simulink model "hoyas_grandes_i_1_sm_computation"  (R2023b)
settings: Solver=FixedStepDiscrete  StartTime=0.0  StopTime=inf  FixedStep=5e-05  RelTol=1e-3  EnableMultiTasking=on
PostLoadFcn:
  | Ts_Power=50e-6;f=50;R_ac=0.12;L_ac=0.08/(2*pi*50);L1=0.17874;L2=0.07596;L3=0.04321;L4=0.01471;L5=0.04751;L6=0.2054;L7=0.17263;L8=0.14418;L9=0.17697;L10=0.19944;L11=0.18905;L12=0.26987;L13=0.1671;L14=0.16874;L15=0.14664;L16=0.12477;L17=0.14989;L18=0.17217;L19=0.19436; load('PV_prof_norm.mat');
InitFcn:
  | Ts_Power=50e-6;f=50;R_ac=0.12;L_ac=0.08/(2*pi*50);L1=0.17874;L2=0.07596;L3=0.04321;L4=0.01471;L5=0.04751;L6=0.2054;L7=0.17263;L8=0.14418;L9=0.17697;L10=0.19944;L11=0.18905;L12=0.26987;L13=0.1671;L14=0.16874;L15=0.14664;L16=0.12477;L17=0.14989;L18=0.17217;L19=0.19436; load('PV_prof_norm.mat');
undefined symbols (not defined in the file or in its folder): D11, Delta, L, X_ac
libraries: spsVoltageMeasurementLib x84, spsCurrentMeasurementLib x75, rtlab x39, spsThreePhaseSeriesRLCBranchLib x38, spsGroundLib x28, powerlib_extras x25, spsThreePhaseDynamicLoadLib x19, eeGeneralControl x4, rteventslib x4, opal_lib x3, spsThreePhasePISectionLineLib x2, spsThreePhaseTransformerTwoWindingsLib x2
(part 1 of 4)
Description:
  | Model of a simple control system for use iin training.
settings Model: Creator=Paul Baracos  LastModifiedBy=depto
settings SolverCC: AlgebraicLoopSolver=TrustRegion
settings DataIOCC: LimitDataPoints=on  SaveFormat=Array  SignalLoggingSaveFormat=ModelDataLogs  SaveOutput=off  SaveTime=off  ReturnWorkspaceOutputs=off  SignalLoggingName=sigsOut
settings OptimizationCC: BlockReduction=off  BooleanDataType=off  OptimizeBlockIOStorage=off  BufferReuse=off  ExpressionFolding=off  LocalBlockOutputs=off  InitFltsAndDblsToZero=on  LifeSpan=inf
settings DebuggingCC: SaveWithParameterizedLinksMsg=none  UnderspecifiedInitializationDetection=Classic  MergeDetectMultiDrivingBlocksExec=none  SignalResolutionControl=TryResolveAllWithWarning  MultiTaskDSMMsg=warning  MultiTaskCondExecSysMsg=none  FcnCallInpInsideContextMsg=warning  UnconnectedInputMsg=warning  UnconnectedOutputMsg=warning  UnconnectedLineMsg=warning  SFUnexpectedBacktrackingDiag=warning  SFNoUnconditionalDefaultTransitionDiag=warning  SFExecutionAtInitializationDiag=none  ArithmeticOperatorsInVariantConditions=warning
settings HardwareCC: ProdBitPerPointer=32  ProdBitPerSizeT=32  ProdBitPerPtrDiffT=32  ProdLargestAtomicFloat=None  ProdIntDivRoundTo=Undefined  ProdEndianess=Unspecified  ProdWordSize=32  ProdHWDeviceType=32-bit Generic  TargetUnknown=on
settings ModelReferenceCC: EnableRefExpFcnMdlSchedulingChecks=on  PropagateSignalLabelsOutOfModel=off
settings SFSimCC: SimUseLocalCustomCode=off  CustomCodeUndefinedFunction=UseInterfaceOnly
settings RTWCC: GenCodeOnly=on  RTWUseLocalCustomCode=off
settings CodeAppCC: StateflowObjectComments=on
settings GRTTargetCC: TargetFcnLib=ansi_tfl_tmw.mat  TargetLangStandard=C89/C90 (ANSI)  CombineOutputUpdateFcns=off  GRTInterface=on
settings ConfigComp: CovMetricSettings=dw  CovSaveCumulativeToWorkspaceVar=on  CovSaveSingleToWorkspaceVar=on  CovExternalEMLEnable=off

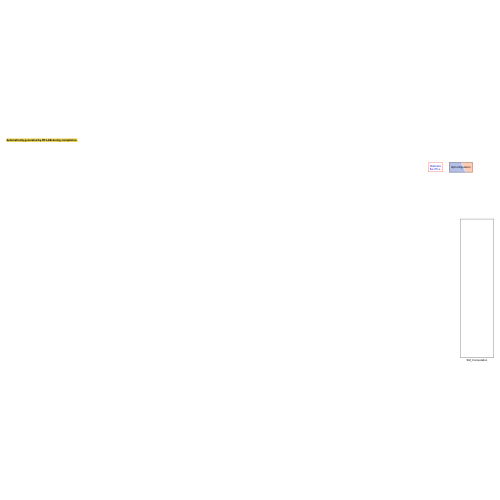
[thumbnail: Simulink's stored preview of the top-level diagram]
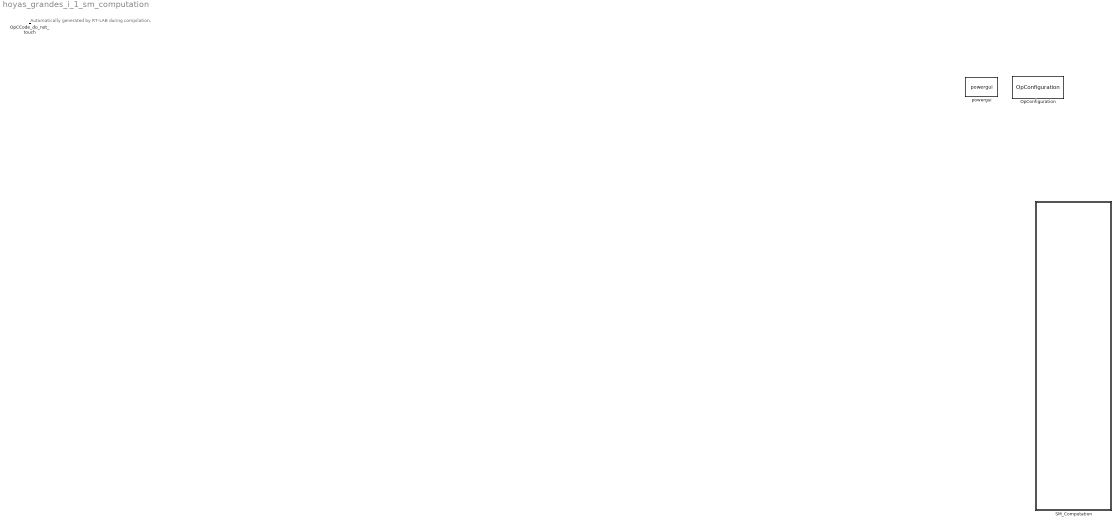
== system hoyas_grandes_i_1_sm_computation ==
  note: Automatically generated by RT-LAB during compilation.
  OpCCode_do_not_touch : opal_lib/Communication/OpCCode  SystemSampleTime=-1  VariantActivationTime=update diagram  AllowFlexibleInterface=on  Latency=0  AutoFrameSizeCalculation=off
  OpConfiguration : rtlab/Miscellaneous/OpConfiguration  Page=Target platform  AddFileBeforeLoad=DatosConstant.mat=binary  AddTargetQnx=off  AddTargetRH=on  AddTargetWin=off  AddTargetPetalinux=on  AddTargetOpalRT=on
      settings: SourceProductName=RT-LAB
  SM_Computation : Subsystem
  powergui : spspowerguiLib/powergui  SimulationMode=Discrete  SampleTime=5e-05  frequency=60  Iterations=50  frequencyindice=50  Pbase=100e6  ErrMax=1e-4  UnitsV=kV  UnitsW=MW  buscounter=0  FunctionMessages=off  echomessages=off  EnableUseOfTLC=off  CurrentSourceSwitches=off  DisableSnubberDevices=off  DisableRonSwitches=off  DisableVfSwitches=off  DisplayEquations=off  AutomaticDiscreteSolvers=off  SolverType=Tustin  Interpol=off  ExternalGateDelay=off  methode=off  Ts=100  x0status=blocks  SPID=off  SwTol=0  HookPort=off  NonlinearTolerance=1e-4  nMaxIteration=100  ContinueOnMaxIteration=off  RestoreLinks=warning  ResistiveCurrentMeasurement=off  Frange=[0:2:500]  Ylog=off  Xlog=on  ShowGrid=off  save=off  variable=ZData  structure=0  ZoomFFT=off  StartTime=0.0  cycles=1  DisplayStyle=1  fundamental=60  FreqAxis=off  MaxFrequency=1000  frequencyindicesteady=1  RmsSteady=1  display=off

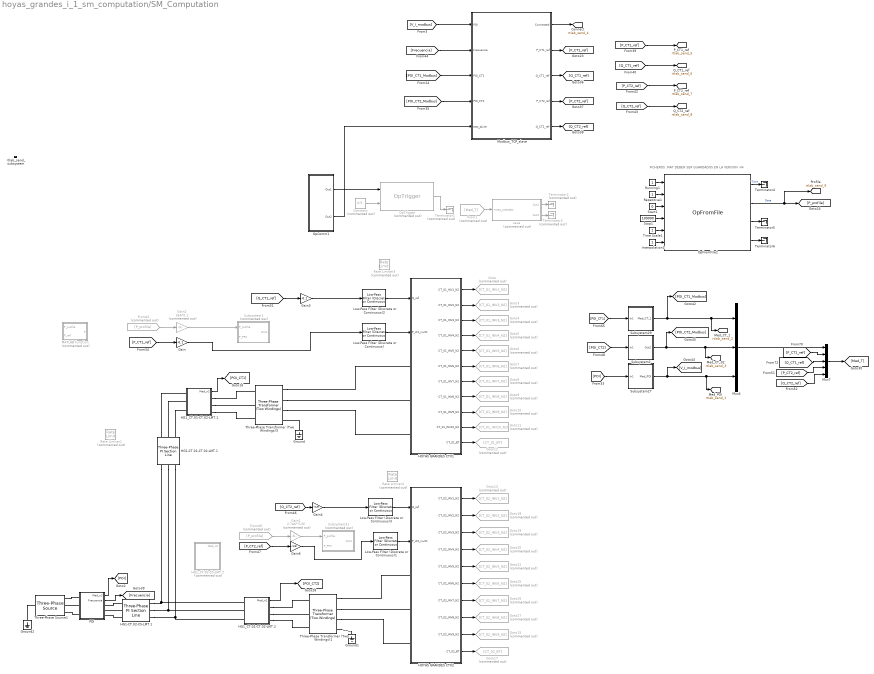
== system hoyas_grandes_i_1_sm_computation/SM_Computation ==
  note: FICHEROS .MAT DEBEN SER GUARDADOS EN LA VERSION -V4
  Constant : Constant  Commented=on  Value=0.5
  From1 : From  Commented=on  GotoTag=Med_T
  From41 : From  Commented=on  GotoTag=P_profile
  From49 : From  Commented=on  GotoTag=P_profile
  Gain : Gain  Gain=-0.1
  Gain1 : Gain  Commented=on  Gain=2.7e6*(1/9)
  Gain2 : Gain  Commented=on  Gain=3e6*0.1
  Gain3 : Gain  Gain=-0.1
  Gain4 : Gain  Gain=-(1/9)
  Gain6 : Gain  Gain=-(1/9)
  Goto : Goto  Commented=on  GotoTag=CT_01_INV1_N2
  Goto10 : Goto  Commented=on  GotoTag=CT_01_INV9_N2
  Goto11 : Goto  Commented=on  GotoTag=CT_01_INV10_N2
  Goto12 : Goto  Commented=on  GotoTag=CT_01_BT
  Goto13 : Goto  Commented=on  GotoTag=CT_02_INV1_N2
  Goto15 : Goto  Commented=on  GotoTag=CT_02_INV9_N2
  Goto17 : Goto  Commented=on  GotoTag=CT_02_BT
  Goto18 : Goto  Commented=on  GotoTag=CT_02_INV2_N2
  Goto19 : Goto  Commented=on  GotoTag=CT_02_INV3_N2
  Goto20 : Goto  Commented=on  GotoTag=CT_02_INV4_N2
  Goto22 : Goto  Commented=on  GotoTag=CT_02_INV5_N2
  Goto25 : Goto  Commented=on  GotoTag=CT_02_INV6_N2
  Goto26 : Goto  Commented=on  GotoTag=CT_02_INV7_N2
  Goto27 : Goto  Commented=on  GotoTag=CT_02_INV8_N2
  Goto3 : Goto  Commented=on  GotoTag=CT_01_INV2_N2
  Goto4 : Goto  Commented=on  GotoTag=CT_01_INV3_N2
  Goto5 : Goto  Commented=on  GotoTag=CT_01_INV4_N2
  Goto6 : Goto  Commented=on  GotoTag=CT_01_INV5_N2
  Goto7 : Goto  Commented=on  GotoTag=CT_01_INV6_N2
  Goto8 : Goto  Commented=on  GotoTag=CT_01_INV7_N2
  Goto9 : Goto  Commented=on  GotoTag=CT_01_INV8_N2
  Ground : spsGroundLib/Ground  LConnTagsString=a
  Ground1 : spsGroundLib/Ground  LConnTagsString=a
  Ground2 : spsGroundLib/Ground  LConnTagsString=a
  HG1-CT.01-CT.02-LMT.1 : spsThreePhasePISectionLineLib/Three-Phase PI Section Line  LConnTagsString=a|b|c  RConnTagsString=A|B|C  Length=0.613  Frequency=50  Resistances=[ 0.206 0.206]  Inductances="[ 0.115/(2*pi*f)  0.115/(2*pi*f)]"  Capacitances=[0.235e-6 0.235e-6]
  HG1-CT.02-CS-LMT.1 : spsThreePhasePISectionLineLib/Three-Phase PI Section Line  LConnTagsString=a|b|c  RConnTagsString=A|B|C  Length=0.153  Frequency=50  Resistances=[ 0.206 0.206]  Inductances="[ 0.115/(2*pi*f)  0.115/(2*pi*f)]"  Capacitances=[0.235e-6 0.235e-6]
  HG1_CT.01-CT.02-LMT.1 : Subsystem
  HG1_CT.01-CT.02-LMT.2 : Subsystem
  HG1_CT.02-CS-LMT.2 : Subsystem  Commented=on
  HOYAS GRANDES CT01 : Subsystem
  HOYAS GRANDES CT02 : Subsystem
  Interpolation1 : Constant
  Low-Pass Filter (Discrete or Continuous){,1..3} (4 alike) : eeGeneralControl/Low-Pass Filter (Discrete or Continuous)  K=1  T=0.03575  B=inf  A=-inf  init_option=Inherited from block input  x0=0  Ts=-1
  MATLAB Function : MATLAB Function  Commented=on  TreatAsAtomicUnit=on
  Modbus_TCP_slave : Subsystem
  Mux4 : Mux  Inputs=3
  Mux7 : Mux  Inputs=5
  OpComm1 : Subsystem
      mask init:
      | opmaskdisplay('maskdisplay_block',gcb,'disp(''OpComm'')');
      mask Display:
      | patch([0 0.5 0.7 0],[1 1 0 0],[0.7 0.75 0.9]);
      | patch([1 0.53 0.73 1],[1 1 0 0],[1 0.8 0.7]);
      | plot([0 0 1 1 0],[0 1 1 0 0]);
      | disp('OpComm')
  OpFromFile2 : rtlab/DataLogging/OpFromFile  filename_mode=Static (same filename all the time)  reload_mode=Next time model is paused (Real-Time)  init_file_id=0  filename=PV_prof_norm.mat  rtpath='./'  nrtpath='.\'  sample_time=0
      settings: SourceProductName=RT-LAB
  OpTrigger : rtlab/DataLogging/OpTrigger  Commented=on  Trig_Type=RISING EDGE  Trig_Offset=0  Acq_Group=28
      settings: SourceProductName=RT-LAB
  POI : Subsystem
  Rate Limiter1 : RateLimiter  Commented=on  RisingSlewLimit=250000*3.5  FallingSlewLimit=-250000*3.5  SampleTimeMode=inherited
  Rate Limiter3 : RateLimiter  Commented=on  RisingSlewLimit=250000*2  FallingSlewLimit=-250000*2  SampleTimeMode=inherited
  Rate Limiter4 : RateLimiter  Commented=on  RisingSlewLimit=250000*2  FallingSlewLimit=-250000*2  SampleTimeMode=inherited
  Repetitive1 : Constant
  Running1 : Constant
  Start1 : Constant  Value=0
  Stop1 : Constant  Value=100000
  Subsystem1 : Subsystem  Commented=on
  Subsystem2 : Subsystem
  Subsystem27 : Subsystem
  Subsystem29 : Subsystem
  Subsystem31 : Subsystem  Commented=on
  Terminator1 : Terminator  Commented=on
  Terminator2 : Terminator  Commented=on
  Terminator3 : Terminator  Commented=on
  Terminator4 : Terminator
  Terminator5 : Terminator
  Terminator6 : Terminator
  Three-Phase Transformer (Two Windings)1 : spsThreePhaseTransformerTwoWindingsLib/Three-Phase Transformer (Two Windings)  Winding1Connection=Delta (D11)  Winding2Connection=Yn  CoreType=Three single-phase transformers  SetSaturation=off  Hysteresis=off  DataFile='hysteresis'  SetInitialFlux=off  Measurements=None  UNITS=pu  NominalPower=[ 3e6 , 50 ]  Winding1=[ 20e3 , 0.0073/2 , 0.0596/2 ]  Winding2=[ 800 , 0.0073/2, 0.0596/2]  Rm=4.7695e3  Lm=4.7695e3  L0=0.5  Saturation=[ 0,0 ; 0.0024,1.2 ; 1.0,1.52 ]  InitialFluxes=[ 0.8 , -0.8 , 0.7 ]  BreakLoop=off  DiscreteSolver=Trapezoidal iterative  DataType=off  TransfoNumber=1
  Three-Phase Transformer (Two Windings)3 : spsThreePhaseTransformerTwoWindingsLib/Three-Phase Transformer (Two Windings)  Winding1Connection=Delta (D11)  Winding2Connection=Yn  CoreType=Three single-phase transformers  SetSaturation=off  Hysteresis=off  DataFile='hysteresis'  SetInitialFlux=off  Measurements=None  UNITS=pu  NominalPower=[ 3e6 , 50 ]  Winding1=[ 20e3 , 0.0073/2 , 0.0596/2 ]  Winding2=[ 800 , 0.0073/2, 0.0596/2]  Rm=4.7695e3  Lm=4.7695e3  L0=0.5  Saturation=[ 0,0 ; 0.0024,1.2 ; 1.0,1.52 ]  InitialFluxes=[ 0.8 , -0.8 , 0.7 ]  BreakLoop=off  DiscreteSolver=Trapezoidal iterative  DataType=off  TransfoNumber=1
  Three-Phase Source1 : spsThreePhaseSourceLib/Three-Phase Source  InternalConnection=Yn  VoltagePhases=off  Voltage=20e3  PhaseAngle=0  Voltage_phases=[25e3 25e3 25e3]/sqrt(3)  PhaseAngles_phases=[0 -120 +120]  Frequency=50  NonIdealSource=on  SpecifyImpedance=on  Resistance=0.8929  Inductance=16.58e-3  ShortCircuitLevel=150.486e6  BaseVoltage=20000  XRratio=3.37  BusType=swing  Pref=10e3  Qref=0  Prefabc=[10e3, 10e3, 10e3]  Qrefabc=[0, 0, 0]  Qmin=-inf  Qmax=inf
  Time Scale1 : Constant
  rtlab_send_subsystem : Subsystem  Priority=-100
      mask Display: text(0,0,'');
  save : Subsystem  Commented=on
  tag scope: rtlab_send_1=global, rtlab_send_2=global, rtlab_send_3=global, rtlab_send_4=global, rtlab_send_5=global, rtlab_send_6=global, rtlab_send_7=global, rtlab_send_8=global, rtlab_send_9=global
  wires:
  [P_CT1_ref] -> Gain/1
  Interpolation1/1 -> OpFromFile2/6
  Repetitive1/1 -> OpFromFile2/2
  HOYAS GRANDES CT02/9(CT_02_INV9_N2) -> Goto15/1
  Gain3/1 -> Low-Pass Filter (Discrete or Continuous)2/1
  OpFromFile2/3 -> Terminator5/1
  Low-Pass Filter (Discrete or Continuous)/1 -> HOYAS GRANDES CT01/2(P_ct1_inv01)
  OpFromFile2/1 -> Terminator4/1  "Time"
  Stop1/1 -> OpFromFile2/4
  HOYAS GRANDES CT01/7(CT_01_INV7_N2) -> Goto8/1
  POI/2(Frecuencia) -> [Frecuencia]
  Running1/1 -> OpFromFile2/1
  [P_CT2_ref] -> Mux7/4
  HOYAS GRANDES CT01/10(CT_01_INV10_N2) -> Goto11/1
  HOYAS GRANDES CT02/8(CT_02_INV8_N2) -> Goto27/1
  OpFromFile2/2 -> [rtlab_send_9], [P_profile]  "Data"
  HG1_CT.01-CT.02-LMT.2/1(Med_n2) -> [POI_CT2]
  OpFromFile2/4 -> Terminator6/1
  HOYAS GRANDES CT01/2(CT_01_INV2_N2) -> Goto3/1
  Start1/1 -> OpFromFile2/3
  [P_CT1_ref] -> Mux7/2
  HOYAS GRANDES CT01/11(CT_01_BT) -> Goto12/1
  HOYAS GRANDES CT02/7(CT_02_INV7_N2) -> Goto26/1
  Time Scale1/1 -> OpFromFile2/5
  Mux7/1 -> [Med_T]
  Subsystem27/1(Med_POI) -> [rtlab_send_1], Mux4/3, [V_I_modbus]
  HOYAS GRANDES CT01/9(CT_01_INV9_N2) -> Goto10/1
  Low-Pass Filter (Discrete or Continuous)1/1 -> HOYAS GRANDES CT02/2(P_ct2_inv01)
  HOYAS GRANDES CT02/2(CT_02_INV2_N2) -> Goto18/1
  HOYAS GRANDES CT01/1(CT_01_INV1_N2) -> Goto/1
  HG1_CT.01-CT.02-LMT.1/1(Med_n2) -> [POI_CT1]
  HOYAS GRANDES CT01/8(CT_01_INV8_N2) -> Goto9/1
  [P_CT2_ref] -> Gain6/1
  From49/1 -> Gain1/1
  HOYAS GRANDES CT01/4(CT_01_INV4_N2) -> Goto5/1
  HOYAS GRANDES CT02/6(CT_02_INV6_N2) -> Goto25/1
  HOYAS GRANDES CT01/5(CT_01_INV5_N2) -> Goto6/1
  HOYAS GRANDES CT02/10(CT_02_BT) -> Goto17/1
  HOYAS GRANDES CT02/5(CT_02_INV5_N2) -> Goto22/1
  HOYAS GRANDES CT02/4(CT_02_INV4_N2) -> Goto20/1
  HOYAS GRANDES CT02/1(CT_02_INV1_N2) -> Goto13/1
  [Q_CT1_ref] -> Mux7/3
  [POI_CT2] -> Subsystem2/1(In1)
  From41/1 -> Gain2/1
  Subsystem2/1(Out2) -> [rtlab_send_3], Mux4/2, [POI_CT2_Modbus]
  Gain4/1 -> Low-Pass Filter (Discrete or Continuous)3/1
  Mux4/1 -> Mux7/1
  HOYAS GRANDES CT01/6(CT_01_INV6_N2) -> Goto7/1
  Subsystem29/1(Med_CT_1) -> [POI_CT1_Modbus], [rtlab_send_2], Mux4/1
  [Q_CT1_ref] -> Gain3/1
  Low-Pass Filter (Discrete or Continuous)2/1 -> HOYAS GRANDES CT01/1(Q_ref)
  [Q_CT2_ref] -> Mux7/5
  [POI_CT1] -> Subsystem29/1(In1)
  POI/1(Med_n2) -> [POI]
  [Q_CT2_ref] -> Gain4/1
  HOYAS GRANDES CT01/3(CT_01_INV3_N2) -> Goto4/1
  OpTrigger/1 -> Terminator1/1
  HOYAS GRANDES CT02/3(CT_02_INV3_N2) -> Goto19/1
  [POI] -> Subsystem27/1(In1)
  Low-Pass Filter (Discrete or Continuous)3/1 -> HOYAS GRANDES CT02/1(Q_ref)
  OpComm1/1(Out1) -> OpTrigger/1
  From1/1 -> save/1(meas_tratadas)
  save/1(Out1) -> Terminator2/1
  Constant/1 -> OpTrigger/2
  save/2(Out2) -> Terminator3/1
  Modbus_TCP_slave/5(Q_CT2_ref) -> [Q_CT2_ref]
  [POI_CT2_Modbus] -> Modbus_TCP_slave/4(POI_CT2)
  Modbus_TCP_slave/3(Q_CT1_ref) -> [Q_CT1_ref]
  [POI_CT1_Modbus] -> Modbus_TCP_slave/3(POI_CT1)
  Modbus_TCP_slave/4(P_CT2_ref) -> [P_CT2_ref]
  Modbus_TCP_slave/1(Connected) -> [rtlab_send_4]
  [V_I_modbus] -> Modbus_TCP_slave/1(POI)
  [Frecuencia] -> Modbus_TCP_slave/2(Frecuencia)
  Modbus_TCP_slave/2(P_CT1_ref) -> [P_CT1_ref]
  [Q_CT2_ref] -> [rtlab_send_8]
  [P_CT2_ref] -> [rtlab_send_7]
  [Q_CT1_ref] -> [rtlab_send_6]
  [P_CT1_ref] -> [rtlab_send_5]
  Gain1/1 -> Subsystem31/1(P_profile)
  Gain6/1 -> Low-Pass Filter (Discrete or Continuous)1/1
  Gain2/1 -> Subsystem1/1(P_profile)
  Gain/1 -> Low-Pass Filter (Discrete or Continuous)/1
  OpComm1/2(Out2) -> Modbus_TCP_slave/5(test_JAvier)
  connections:
  Three-Phase Transformer (Two Windings)1/RConn4 -- Ground1/LConn1
  HG1-CT.01-CT.02-LMT.1/RConn3 -- HG1_CT.01-CT.02-LMT.1/LConn3
  Ground/LConn1 -- Three-Phase Transformer (Two Windings)3/RConn4
  Three-Phase Transformer (Two Windings)3/RConn3 -- HOYAS GRANDES CT01/LConn3
  Three-Phase Transformer (Two Windings)1/RConn3 -- HOYAS GRANDES CT02/LConn3
  HG1-CT.01-CT.02-LMT.1/RConn2 -- HG1_CT.01-CT.02-LMT.1/LConn2
  HG1-CT.02-CS-LMT.1/LConn1 -- POI/RConn1
  HG1_CT.01-CT.02-LMT.1/RConn3 -- Three-Phase Transformer (Two Windings)3/LConn3
  POI/LConn1 -- Three-Phase Source1/RConn1
  Three-Phase Transformer (Two Windings)3/RConn2 -- HOYAS GRANDES CT01/LConn2
  Three-Phase Transformer (Two Windings)1/RConn1 -- HOYAS GRANDES CT02/LConn1
  HG1_CT.01-CT.02-LMT.2/RConn2 -- Three-Phase Transformer (Two Windings)1/LConn2
  HG1_CT.01-CT.02-LMT.1/RConn2 -- Three-Phase Transformer (Two Windings)3/LConn2
  HG1-CT.02-CS-LMT.1/RConn3 -- HG1_CT.01-CT.02-LMT.2/LConn3 -- HG1-CT.01-CT.02-LMT.1/LConn3
  HG1_CT.01-CT.02-LMT.2/RConn1 -- Three-Phase Transformer (Two Windings)1/LConn1
  HG1-CT.02-CS-LMT.1/RConn1 -- HG1_CT.01-CT.02-LMT.2/LConn1 -- HG1-CT.01-CT.02-LMT.1/LConn1
  HG1-CT.02-CS-LMT.1/RConn2 -- HG1_CT.01-CT.02-LMT.2/LConn2 -- HG1-CT.01-CT.02-LMT.1/LConn2
  Three-Phase Transformer (Two Windings)3/RConn1 -- HOYAS GRANDES CT01/LConn1
  Ground2/LConn1 -- Three-Phase Source1/LConn1
  HG1-CT.02-CS-LMT.1/LConn3 -- POI/RConn3
  HG1_CT.01-CT.02-LMT.2/RConn3 -- Three-Phase Transformer (Two Windings)1/LConn3
  POI/LConn2 -- Three-Phase Source1/RConn2
  POI/LConn3 -- Three-Phase Source1/RConn3
  HG1_CT.01-CT.02-LMT.1/RConn1 -- Three-Phase Transformer (Two Windings)3/LConn1
  HG1-CT.02-CS-LMT.1/LConn2 -- POI/RConn2
  HG1-CT.01-CT.02-LMT.1/RConn1 -- HG1_CT.01-CT.02-LMT.1/LConn1
  Three-Phase Transformer (Two Windings)1/RConn2 -- HOYAS GRANDES CT02/LConn2

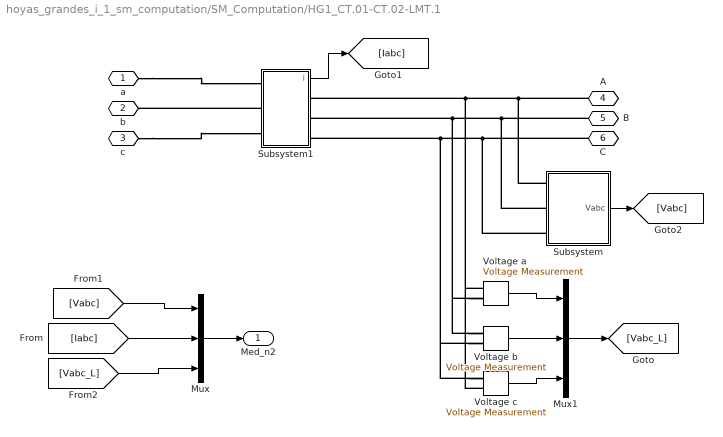
== system hoyas_grandes_i_1_sm_computation/SM_Computation/HG1_CT.01-CT.02-LMT.1 ==
  Mux : Mux  Inputs=3
  Mux1 : Mux  Inputs=3
  Subsystem : Subsystem
  Subsystem1 : Subsystem
  Voltage a : spsVoltageMeasurementLib/Voltage Measurement  PhasorSimulation=off  OutputType=Complex  PSBequivalent=0
  Voltage b : spsVoltageMeasurementLib/Voltage Measurement  PhasorSimulation=off  OutputType=Complex  PSBequivalent=0
  Voltage c : spsVoltageMeasurementLib/Voltage Measurement  PhasorSimulation=off  OutputType=Complex  PSBequivalent=0
  a : PMIOPort  Side=Right
  b : PMIOPort  Port=2  Side=Right
  c : PMIOPort  Port=3  Side=Right
  A : PMIOPort  Port=4  Side=Left
  B : PMIOPort  Port=5  Side=Left
  C : PMIOPort  Port=6  Side=Left
  Med_n2 : Outport
  wires:
  Subsystem1/1(i) -> [Iabc]
  [Vabc] -> Mux/1
  [Iabc] -> Mux/2
  Mux/1 -> Med_n2/1
  Voltage a/1 -> Mux1/1
  Voltage b/1 -> Mux1/2
  Voltage c/1 -> Mux1/3
  Mux1/1 -> [Vabc_L]
  Subsystem/1(Vabc) -> [Vabc]
  [Vabc_L] -> Mux/3
  connections:
  B/RConn1 -- Subsystem/LConn2 -- Voltage b/LConn1 -- Voltage a/LConn2 -- Subsystem1/RConn2
  A/RConn1 -- Subsystem/LConn1 -- Voltage a/LConn1 -- Voltage c/LConn2 -- Subsystem1/RConn1
  C/RConn1 -- Subsystem/LConn3 -- Voltage c/LConn1 -- Voltage b/LConn2 -- Subsystem1/RConn3
  c/RConn1 -- Subsystem1/LConn3
  Subsystem1/LConn2 -- b/RConn1
  a/RConn1 -- Subsystem1/LConn1

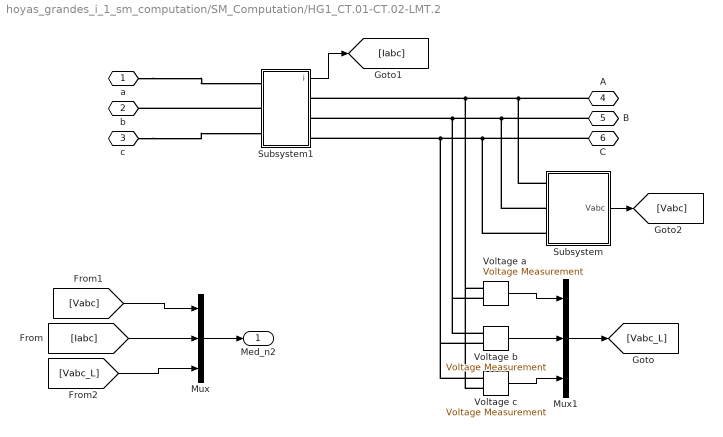
== system hoyas_grandes_i_1_sm_computation/SM_Computation/HG1_CT.01-CT.02-LMT.2 ==
  Mux : Mux  Inputs=3
  Mux1 : Mux  Inputs=3
  Subsystem : Subsystem
  Subsystem1 : Subsystem
  Voltage a : spsVoltageMeasurementLib/Voltage Measurement  PhasorSimulation=off  OutputType=Complex  PSBequivalent=0
  Voltage b : spsVoltageMeasurementLib/Voltage Measurement  PhasorSimulation=off  OutputType=Complex  PSBequivalent=0
  Voltage c : spsVoltageMeasurementLib/Voltage Measurement  PhasorSimulation=off  OutputType=Complex  PSBequivalent=0
  a : PMIOPort  Side=Right
  b : PMIOPort  Port=2  Side=Right
  c : PMIOPort  Port=3  Side=Right
  A : PMIOPort  Port=4  Side=Left
  B : PMIOPort  Port=5  Side=Left
  C : PMIOPort  Port=6  Side=Left
  Med_n2 : Outport
  wires:
  [Vabc_L] -> Mux/3
  Subsystem/1(Vabc) -> [Vabc]
  Mux1/1 -> [Vabc_L]
  Voltage c/1 -> Mux1/3
  Voltage b/1 -> Mux1/2
  Voltage a/1 -> Mux1/1
  Mux/1 -> Med_n2/1
  [Iabc] -> Mux/2
  [Vabc] -> Mux/1
  Subsystem1/1(i) -> [Iabc]
  connections:
  a/RConn1 -- Subsystem1/LConn1
  Subsystem1/LConn2 -- b/RConn1
  c/RConn1 -- Subsystem1/LConn3
  Subsystem/LConn3 -- C/RConn1 -- Subsystem1/RConn3 -- Voltage b/LConn2 -- Voltage c/LConn1
  Subsystem/LConn1 -- A/RConn1 -- Subsystem1/RConn1 -- Voltage c/LConn2 -- Voltage a/LConn1
  Subsystem/LConn2 -- B/RConn1 -- Subsystem1/RConn2 -- Voltage a/LConn2 -- Voltage b/LConn1

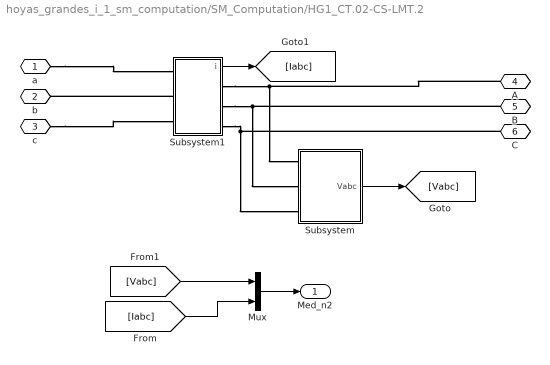
== system hoyas_grandes_i_1_sm_computation/SM_Computation/HG1_CT.02-CS-LMT.2 ==
  Mux : Mux  Inputs=2
  Subsystem : Subsystem
  Subsystem1 : Subsystem
  a : PMIOPort  Side=Right
  b : PMIOPort  Port=2  Side=Right
  c : PMIOPort  Port=3  Side=Right
  A : PMIOPort  Port=4  Side=Left
  B : PMIOPort  Port=5  Side=Left
  C : PMIOPort  Port=6  Side=Left
  Med_n2 : Outport
  wires:
  Subsystem/1(Vabc) -> [Vabc]
  Subsystem1/1(i) -> [Iabc]
  [Vabc] -> Mux/1
  [Iabc] -> Mux/2
  Mux/1 -> Med_n2/1
  connections:
  Subsystem1/RConn2 -- B/RConn1 -- Subsystem/LConn2
  Subsystem1/RConn1 -- A/RConn1 -- Subsystem/LConn1
  Subsystem1/RConn3 -- C/RConn1 -- Subsystem/LConn3
  c/RConn1 -- Subsystem1/LConn3
  Subsystem1/LConn2 -- b/RConn1
  a/RConn1 -- Subsystem1/LConn1

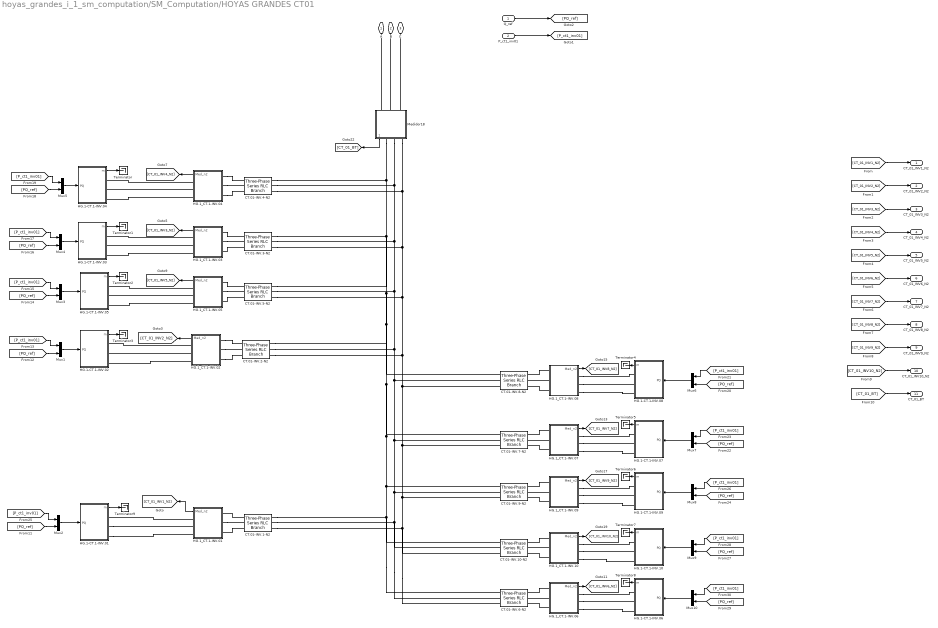
== system hoyas_grandes_i_1_sm_computation/SM_Computation/HOYAS GRANDES CT01 ==
  Q_ref : Inport
  P_ct1_inv01 : Inport  Port=2
  CT.01-INV.1-N2 : spsThreePhaseSeriesRLCBranchLib/Three-Phase Series RLC Branch  LConnTagsString=A|B|C  RConnTagsString=A|B|C  BranchType=RL  Resistance=R_ac*L1  Inductance=L_ac*L1  Capacitance=1e-6  Measurements=None
  CT.01-INV.10-N2 : spsThreePhaseSeriesRLCBranchLib/Three-Phase Series RLC Branch  LConnTagsString=A|B|C  RConnTagsString=A|B|C  BranchType=RL  Resistance=R_ac*L10  Inductance=L_ac*L10  Capacitance=1e-6  Measurements=None
  CT.01-INV.2-N2 : spsThreePhaseSeriesRLCBranchLib/Three-Phase Series RLC Branch  LConnTagsString=A|B|C  RConnTagsString=A|B|C  BranchType=RL  Resistance=R_ac*L2  Inductance=L_ac*L2  Capacitance=1e-6  Measurements=None
  CT.01-INV.3-N2 : spsThreePhaseSeriesRLCBranchLib/Three-Phase Series RLC Branch  LConnTagsString=A|B|C  RConnTagsString=A|B|C  BranchType=RL  Resistance=R_ac*L3  Inductance=L_ac*L3  Capacitance=1e-6  Measurements=None
  CT.01-INV.4-N2 : spsThreePhaseSeriesRLCBranchLib/Three-Phase Series RLC Branch  LConnTagsString=A|B|C  RConnTagsString=A|B|C  BranchType=RL  Resistance=R_ac*L4  Inductance=L_ac*L4  Capacitance=1e-6  Measurements=None
  CT.01-INV.5-N2 : spsThreePhaseSeriesRLCBranchLib/Three-Phase Series RLC Branch  LConnTagsString=A|B|C  RConnTagsString=A|B|C  BranchType=RL  Resistance=R_ac*L5  Inductance=L_ac*L5  Capacitance=1e-6  Measurements=None
  CT.01-INV.6-N2 : spsThreePhaseSeriesRLCBranchLib/Three-Phase Series RLC Branch  LConnTagsString=A|B|C  RConnTagsString=A|B|C  BranchType=RL  Resistance=R_ac*L6  Inductance=L_ac*L6  Capacitance=1e-6  Measurements=None
  CT.01-INV.7-N2 : spsThreePhaseSeriesRLCBranchLib/Three-Phase Series RLC Branch  LConnTagsString=A|B|C  RConnTagsString=A|B|C  BranchType=RL  Resistance=R_ac*L7  Inductance=L_ac*L7  Capacitance=1e-6  Measurements=None
  CT.01-INV.8-N2 : spsThreePhaseSeriesRLCBranchLib/Three-Phase Series RLC Branch  LConnTagsString=A|B|C  RConnTagsString=A|B|C  BranchType=RL  Resistance=R_ac*L8  Inductance=L_ac*L8  Capacitance=1e-6  Measurements=None
  CT.01-INV.9-N2 : spsThreePhaseSeriesRLCBranchLib/Three-Phase Series RLC Branch  LConnTagsString=A|B|C  RConnTagsString=A|B|C  BranchType=RL  Resistance=R_ac*L9  Inductance=L_ac*L9  Capacitance=1e-6  Measurements=None
  HG.1-CT.1-INV.01 : Subsystem
  HG.1-CT.1-INV.02 : Subsystem
  HG.1-CT.1-INV.03 : Subsystem
  HG.1-CT.1-INV.04 : Subsystem
  HG.1-CT.1-INV.05 : Subsystem
  HG.1-CT.1-INV.06 : Subsystem
  HG.1-CT.1-INV.07 : Subsystem
  HG.1-CT.1-INV.08 : Subsystem
  HG.1-CT.1-INV.09 : Subsystem
  HG.1-CT.1-INV.10 : Subsystem
  HG.1_CT.1-INV.01 : Subsystem
  HG.1_CT.1-INV.02 : Subsystem
  HG.1_CT.1-INV.03 : Subsystem
  HG.1_CT.1-INV.04 : Subsystem
  HG.1_CT.1-INV.05 : Subsystem
  HG.1_CT.1-INV.06 : Subsystem
  HG.1_CT.1-INV.07 : Subsystem
  HG.1_CT.1-INV.08 : Subsystem
  HG.1_CT.1-INV.09 : Subsystem
  HG.1_CT.1-INV.10 : Subsystem
  Medidor18 : Subsystem
  Mux{1..10} (10 alike) : Mux  Inputs=2
  Terminator{,1..9} (10 alike) : Terminator
  A : PMIOPort  Side=Left
  B : PMIOPort  Port=2  Side=Left
  C : PMIOPort  Port=3  Side=Left
  CT_01_INV1_N2 : Outport
  CT_01_INV2_N2 : Outport  Port=2
  CT_01_INV3_N2 : Outport  Port=3
  CT_01_INV4_N2 : Outport  Port=4
  CT_01_INV5_N2 : Outport  Port=5
  CT_01_INV6_N2 : Outport  Port=6
  CT_01_INV7_N2 : Outport  Port=7
  CT_01_INV8_N2 : Outport  Port=8
  CT_01_INV9_N2 : Outport  Port=9
  CT_01_INV10_N2 : Outport  Port=10
  CT_01_BT : Outport  Port=11
  wires:
  Medidor18/1(Med_n2) -> [CT_01_BT]
  HG.1_CT.1-INV.06/1(Med_n2) -> [CT_01_INV6_N2]
  HG.1_CT.1-INV.01/1(Med_n2) -> [CT_01_INV1_N2]
  HG.1_CT.1-INV.05/1(Med_n2) -> [CT_01_INV5_N2]
  HG.1_CT.1-INV.04/1(Med_n2) -> [CT_01_INV4_N2]
  HG.1_CT.1-INV.09/1(Med_n2) -> [CT_01_INV9_N2]
  HG.1_CT.1-INV.07/1(Med_n2) -> [CT_01_INV7_N2]
  HG.1_CT.1-INV.02/1(Med_n2) -> [CT_01_INV2_N2]
  HG.1_CT.1-INV.03/1(Med_n2) -> [CT_01_INV3_N2]
  HG.1_CT.1-INV.08/1(Med_n2) -> [CT_01_INV8_N2]
  HG.1_CT.1-INV.10/1(Med_n2) -> [CT_01_INV10_N2]
  P_ct1_inv01/1 -> [P_ct1_inv01]
  [CT_01_INV1_N2] -> CT_01_INV1_N2/1
  [CT_01_BT] -> CT_01_BT/1
  [P_ct1_inv01] -> Mux2/1
  [CT_01_INV2_N2] -> CT_01_INV2_N2/1
  [CT_01_INV3_N2] -> CT_01_INV3_N2/1
  [CT_01_INV5_N2] -> CT_01_INV5_N2/1
  [CT_01_INV4_N2] -> CT_01_INV4_N2/1
  [CT_01_INV6_N2] -> CT_01_INV6_N2/1
  [CT_01_INV7_N2] -> CT_01_INV7_N2/1
  [CT_01_INV8_N2] -> CT_01_INV8_N2/1
  [CT_01_INV9_N2] -> CT_01_INV9_N2/1
  [CT_01_INV10_N2] -> CT_01_INV10_N2/1
  HG.1-CT.1-INV.04/1(m) -> Terminator/1
  HG.1-CT.1-INV.03/1(m) -> Terminator1/1
  HG.1-CT.1-INV.05/1(m) -> Terminator2/1
  HG.1-CT.1-INV.02/1(m) -> Terminator3/1
  HG.1-CT.1-INV.08/1(m) -> Terminator4/1
  HG.1-CT.1-INV.07/1(m) -> Terminator5/1
  HG.1-CT.1-INV.09/1(m) -> Terminator6/1
  HG.1-CT.1-INV.10/1(m) -> Terminator7/1
  HG.1-CT.1-INV.06/1(m) -> Terminator8/1
  Mux2/1 -> HG.1-CT.1-INV.01/1(PQ)
  [PQ_ref] -> Mux2/2
  Q_ref/1 -> [PQ_ref]
  [PQ_ref] -> Mux1/2
  Mux1/1 -> HG.1-CT.1-INV.02/1(PQ)
  [P_ct1_inv01] -> Mux1/1
  [P_ct1_inv01] -> Mux3/1
  Mux3/1 -> HG.1-CT.1-INV.05/1(PQ)
  [PQ_ref] -> Mux3/2
  [PQ_ref] -> Mux4/2
  Mux4/1 -> HG.1-CT.1-INV.03/1(PQ)
  [P_ct1_inv01] -> Mux4/1
  [P_ct1_inv01] -> Mux5/1
  Mux5/1 -> HG.1-CT.1-INV.04/1(PQ)
  [PQ_ref] -> Mux5/2
  [PQ_ref] -> Mux6/2
  [P_ct1_inv01] -> Mux6/1
  Mux6/1 -> HG.1-CT.1-INV.08/1(PQ)
  Mux7/1 -> HG.1-CT.1-INV.07/1(PQ)
  [P_ct1_inv01] -> Mux7/1
  [PQ_ref] -> Mux7/2
  [PQ_ref] -> Mux8/2
  [P_ct1_inv01] -> Mux8/1
  Mux8/1 -> HG.1-CT.1-INV.09/1(PQ)
  Mux9/1 -> HG.1-CT.1-INV.10/1(PQ)
  [P_ct1_inv01] -> Mux9/1
  [PQ_ref] -> Mux9/2
  [PQ_ref] -> Mux10/2
  [P_ct1_inv01] -> Mux10/1
  Mux10/1 -> HG.1-CT.1-INV.06/1(PQ)
  HG.1-CT.1-INV.01/1(m) -> Terminator9/1
  connections:
  HG.1_CT.1-INV.09/LConn1 -- CT.01-INV.9-N2/RConn1
  HG.1_CT.1-INV.07/RConn1 -- HG.1-CT.1-INV.07/RConn1
  HG.1_CT.1-INV.06/LConn3 -- CT.01-INV.6-N2/RConn3
  HG.1_CT.1-INV.08/RConn3 -- HG.1-CT.1-INV.08/RConn3
  HG.1_CT.1-INV.04/LConn1 -- CT.01-INV.4-N2/RConn1
  HG.1_CT.1-INV.06/RConn3 -- HG.1-CT.1-INV.06/RConn3
  HG.1_CT.1-INV.06/LConn1 -- CT.01-INV.6-N2/RConn1
  HG.1_CT.1-INV.08/RConn1 -- HG.1-CT.1-INV.08/RConn1
  HG.1_CT.1-INV.02/LConn3 -- CT.01-INV.2-N2/RConn3
  HG.1_CT.1-INV.07/LConn1 -- CT.01-INV.7-N2/RConn1
  HG.1_CT.1-INV.10/LConn1 -- CT.01-INV.10-N2/RConn1
  HG.1_CT.1-INV.05/LConn3 -- CT.01-INV.5-N2/RConn3
  HG.1_CT.1-INV.03/RConn2 -- HG.1-CT.1-INV.03/RConn2
  HG.1_CT.1-INV.05/RConn1 -- HG.1-CT.1-INV.05/RConn1
  HG.1_CT.1-INV.03/LConn3 -- CT.01-INV.3-N2/RConn3
  Medidor18/LConn3 -- C/RConn1
  HG.1_CT.1-INV.09/LConn3 -- CT.01-INV.9-N2/RConn3
  Medidor18/RConn3 -- CT.01-INV.4-N2/LConn3 -- CT.01-INV.5-N2/LConn3 -- CT.01-INV.2-N2/LConn3 -- CT.01-INV.8-N2/LConn3 -- CT.01-INV.6-N2/LConn3 -- CT.01-INV.10-N2/LConn3 -- CT.01-INV.1-N2/LConn3 -- CT.01-INV.9-N2/LConn3 -- CT.01-INV.7-N2/LConn3 -- CT.01-INV.3-N2/LConn3
  HG.1_CT.1-INV.08/LConn2 -- CT.01-INV.8-N2/RConn2
  HG.1_CT.1-INV.05/RConn2 -- HG.1-CT.1-INV.05/RConn2
  HG.1_CT.1-INV.03/RConn1 -- HG.1-CT.1-INV.03/RConn1
  HG.1_CT.1-INV.02/LConn2 -- CT.01-INV.2-N2/RConn2
  HG.1_CT.1-INV.03/LConn2 -- CT.01-INV.3-N2/RConn2
  HG.1_CT.1-INV.04/RConn1 -- HG.1-CT.1-INV.04/RConn1
  HG.1_CT.1-INV.04/RConn3 -- HG.1-CT.1-INV.04/RConn3
  HG.1_CT.1-INV.09/RConn2 -- HG.1-CT.1-INV.09/RConn2
  Medidor18/RConn1 -- CT.01-INV.4-N2/LConn1 -- CT.01-INV.2-N2/LConn1 -- CT.01-INV.8-N2/LConn1 -- CT.01-INV.7-N2/LConn1 -- CT.01-INV.6-N2/LConn1 -- CT.01-INV.10-N2/LConn1 -- CT.01-INV.1-N2/LConn1 -- CT.01-INV.9-N2/LConn1 -- CT.01-INV.5-N2/LConn1 -- CT.01-INV.3-N2/LConn1
  HG.1_CT.1-INV.03/RConn3 -- HG.1-CT.1-INV.03/RConn3
  HG.1_CT.1-INV.01/LConn2 -- CT.01-INV.1-N2/RConn2
  HG.1_CT.1-INV.09/RConn3 -- HG.1-CT.1-INV.09/RConn3
  HG.1_CT.1-INV.07/LConn3 -- CT.01-INV.7-N2/RConn3
  HG.1_CT.1-INV.07/RConn2 -- HG.1-CT.1-INV.07/RConn2
  HG.1_CT.1-INV.05/LConn1 -- CT.01-INV.5-N2/RConn1
  HG.1_CT.1-INV.07/LConn2 -- CT.01-INV.7-N2/RConn2
  HG.1_CT.1-INV.08/LConn3 -- CT.01-INV.8-N2/RConn3
  HG.1_CT.1-INV.08/LConn1 -- CT.01-INV.8-N2/RConn1
  HG.1-CT.1-INV.01/RConn3 -- HG.1_CT.1-INV.01/RConn3
  HG.1_CT.1-INV.10/RConn2 -- HG.1-CT.1-INV.10/RConn2
  HG.1_CT.1-INV.09/RConn1 -- HG.1-CT.1-INV.09/RConn1
  CT.01-INV.1-N2/RConn3 -- HG.1_CT.1-INV.01/LConn3
  HG.1_CT.1-INV.04/LConn3 -- CT.01-INV.4-N2/RConn3
  HG.1_CT.1-INV.03/LConn1 -- CT.01-INV.3-N2/RConn1
  HG.1_CT.1-INV.10/LConn2 -- CT.01-INV.10-N2/RConn2
  HG.1_CT.1-INV.06/RConn1 -- HG.1-CT.1-INV.06/RConn1
  HG.1_CT.1-INV.09/LConn2 -- CT.01-INV.9-N2/RConn2
  HG.1_CT.1-INV.04/LConn2 -- CT.01-INV.4-N2/RConn2
  HG.1_CT.1-INV.10/RConn3 -- HG.1-CT.1-INV.10/RConn3
  HG.1_CT.1-INV.05/RConn3 -- HG.1-CT.1-INV.05/RConn3
  HG.1_CT.1-INV.04/RConn2 -- HG.1-CT.1-INV.04/RConn2
  HG.1_CT.1-INV.01/RConn1 -- HG.1-CT.1-INV.01/RConn1
  HG.1_CT.1-INV.10/LConn3 -- CT.01-INV.10-N2/RConn3
  HG.1_CT.1-INV.02/LConn1 -- CT.01-INV.2-N2/RConn1
  CT.01-INV.1-N2/RConn1 -- HG.1_CT.1-INV.01/LConn1
  Medidor18/RConn2 -- CT.01-INV.4-N2/LConn2 -- CT.01-INV.5-N2/LConn2 -- CT.01-INV.8-N2/LConn2 -- CT.01-INV.6-N2/LConn2 -- CT.01-INV.10-N2/LConn2 -- CT.01-INV.1-N2/LConn2 -- CT.01-INV.9-N2/LConn2 -- CT.01-INV.7-N2/LConn2 -- CT.01-INV.2-N2/LConn2 -- CT.01-INV.3-N2/LConn2
  HG.1_CT.1-INV.10/RConn1 -- HG.1-CT.1-INV.10/RConn1
  HG.1_CT.1-INV.05/LConn2 -- CT.01-INV.5-N2/RConn2
  HG.1_CT.1-INV.07/RConn3 -- HG.1-CT.1-INV.07/RConn3
  HG.1_CT.1-INV.08/RConn2 -- HG.1-CT.1-INV.08/RConn2
  HG.1_CT.1-INV.06/LConn2 -- CT.01-INV.6-N2/RConn2
  HG.1-CT.1-INV.01/RConn2 -- HG.1_CT.1-INV.01/RConn2
  HG.1_CT.1-INV.06/RConn2 -- HG.1-CT.1-INV.06/RConn2
  Medidor18/LConn2 -- B/RConn1
  Medidor18/LConn1 -- A/RConn1
  HG.1_CT.1-INV.02/RConn1 -- HG.1-CT.1-INV.02/RConn1
  HG.1_CT.1-INV.02/RConn2 -- HG.1-CT.1-INV.02/RConn2
  HG.1_CT.1-INV.02/RConn3 -- HG.1-CT.1-INV.02/RConn3

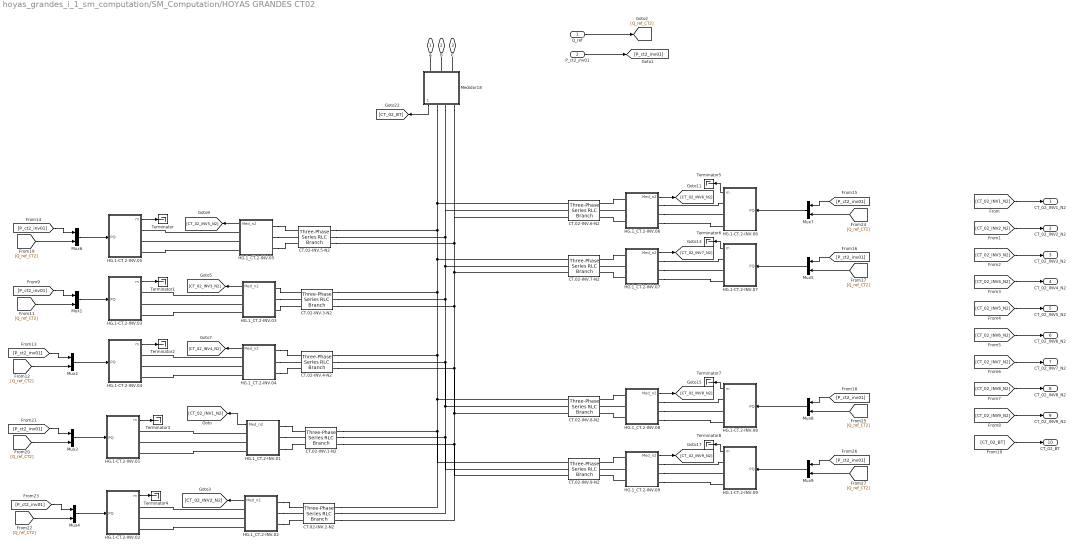
== system hoyas_grandes_i_1_sm_computation/SM_Computation/HOYAS GRANDES CT02 ==
  Q_ref : Inport
  P_ct2_inv01 : Inport  Port=2
  CT.02-INV.1-N2 : spsThreePhaseSeriesRLCBranchLib/Three-Phase Series RLC Branch  LConnTagsString=A|B|C  RConnTagsString=A|B|C  BranchType=RL  Resistance=R_ac*L11  Inductance=L_ac*L11  Capacitance=1e-6  Measurements=None
  CT.02-INV.2-N2 : spsThreePhaseSeriesRLCBranchLib/Three-Phase Series RLC Branch  LConnTagsString=A|B|C  RConnTagsString=A|B|C  BranchType=RL  Resistance=0.09*L12  Inductance=L_ac*L12  Capacitance=1e-6  Measurements=None
  CT.02-INV.3-N2 : spsThreePhaseSeriesRLCBranchLib/Three-Phase Series RLC Branch  LConnTagsString=A|B|C  RConnTagsString=A|B|C  BranchType=RL  Resistance=R_ac*L13  Inductance=L_ac*L13  Capacitance=1e-6  Measurements=None
  CT.02-INV.4-N2 : spsThreePhaseSeriesRLCBranchLib/Three-Phase Series RLC Branch  LConnTagsString=A|B|C  RConnTagsString=A|B|C  BranchType=RL  Resistance=R_ac*L14  Inductance=L_ac*L14  Capacitance=1e-6  Measurements=None
  CT.02-INV.5-N2 : spsThreePhaseSeriesRLCBranchLib/Three-Phase Series RLC Branch  LConnTagsString=A|B|C  RConnTagsString=A|B|C  BranchType=RL  Resistance=R_ac*L15  Inductance=L_ac*L15  Capacitance=1e-6  Measurements=None
  CT.02-INV.6-N2 : spsThreePhaseSeriesRLCBranchLib/Three-Phase Series RLC Branch  LConnTagsString=A|B|C  RConnTagsString=A|B|C  BranchType=RL  Resistance=R_ac*L16  Inductance=L_ac*L16  Capacitance=1e-6  Measurements=None
  CT.02-INV.7-N2 : spsThreePhaseSeriesRLCBranchLib/Three-Phase Series RLC Branch  LConnTagsString=A|B|C  RConnTagsString=A|B|C  BranchType=RL  Resistance=R_ac*L17  Inductance=L_ac*L17  Capacitance=1e-6  Measurements=None
  CT.02-INV.8-N2 : spsThreePhaseSeriesRLCBranchLib/Three-Phase Series RLC Branch  LConnTagsString=A|B|C  RConnTagsString=A|B|C  BranchType=RL  Resistance=R_ac*L18  Inductance=L_ac*L18  Capacitance=1e-6  Measurements=None
  CT.02-INV.9-N2 : spsThreePhaseSeriesRLCBranchLib/Three-Phase Series RLC Branch  LConnTagsString=A|B|C  RConnTagsString=A|B|C  BranchType=RL  Resistance=R_ac*L19  Inductance=L_ac*L19  Capacitance=1e-6  Measurements=None
  HG.1-CT.2-INV.01 : Subsystem
  HG.1-CT.2-INV.02 : Subsystem
  HG.1-CT.2-INV.03 : Subsystem
  HG.1-CT.2-INV.04 : Subsystem
  HG.1-CT.2-INV.05 : Subsystem
  HG.1-CT.2-INV.06 : Subsystem
  HG.1-CT.2-INV.07 : Subsystem
  HG.1-CT.2-INV.08 : Subsystem
  HG.1-CT.2-INV.09 : Subsystem
  HG.1_CT.2-INV.01 : Subsystem
  HG.1_CT.2-INV.02 : Subsystem
  HG.1_CT.2-INV.03 : Subsystem
  HG.1_CT.2-INV.04 : Subsystem
  HG.1_CT.2-INV.05 : Subsystem
  HG.1_CT.2-INV.06 : Subsystem
  HG.1_CT.2-INV.07 : Subsystem
  HG.1_CT.2-INV.08 : Subsystem
  HG.1_CT.2-INV.09 : Subsystem
  Medidor18 : Subsystem
  Mux{1..9} (9 alike) : Mux  Inputs=2
  Terminator{,1..8} (9 alike) : Terminator
  A : PMIOPort  Side=Left
  B : PMIOPort  Port=2  Side=Left
  C : PMIOPort  Port=3  Side=Left
  CT_02_INV1_N2 : Outport
  CT_02_INV2_N2 : Outport  Port=2
  CT_02_INV3_N2 : Outport  Port=3
  CT_02_INV4_N2 : Outport  Port=4
  CT_02_INV5_N2 : Outport  Port=5
  CT_02_INV6_N2 : Outport  Port=6
  CT_02_INV7_N2 : Outport  Port=7
  CT_02_INV8_N2 : Outport  Port=8
  CT_02_INV9_N2 : Outport  Port=9
  CT_02_BT : Outport  Port=10
  wires:
  [CT_02_BT] -> CT_02_BT/1
  [CT_02_INV9_N2] -> CT_02_INV9_N2/1
  [CT_02_INV8_N2] -> CT_02_INV8_N2/1
  [CT_02_INV7_N2] -> CT_02_INV7_N2/1
  [CT_02_INV6_N2] -> CT_02_INV6_N2/1
  [CT_02_INV5_N2] -> CT_02_INV5_N2/1
  [CT_02_INV4_N2] -> CT_02_INV4_N2/1
  [CT_02_INV3_N2] -> CT_02_INV3_N2/1
  [CT_02_INV2_N2] -> CT_02_INV2_N2/1
  [CT_02_INV1_N2] -> CT_02_INV1_N2/1
  P_ct2_inv01/1 -> [P_ct2_inv01]
  Mux6/1 -> HG.1-CT.2-INV.05/1(PQ)
  [Q_ref_CT2] -> Mux7/2
  [P_ct2_inv01] -> Mux6/1
  [P_ct2_inv01] -> Mux7/1
  [Q_ref_CT2] -> Mux6/2
  Mux7/1 -> HG.1-CT.2-INV.06/1(PQ)
  HG.1_CT.2-INV.08/1(Med_n2) -> [CT_02_INV8_N2]
  HG.1_CT.2-INV.03/1(Med_n2) -> [CT_02_INV3_N2]
  HG.1_CT.2-INV.02/1(Med_n2) -> [CT_02_INV2_N2]
  HG.1_CT.2-INV.07/1(Med_n2) -> [CT_02_INV7_N2]
  HG.1_CT.2-INV.09/1(Med_n2) -> [CT_02_INV9_N2]
  HG.1_CT.2-INV.04/1(Med_n2) -> [CT_02_INV4_N2]
  HG.1_CT.2-INV.05/1(Med_n2) -> [CT_02_INV5_N2]
  HG.1_CT.2-INV.01/1(Med_n2) -> [CT_02_INV1_N2]
  HG.1_CT.2-INV.06/1(Med_n2) -> [CT_02_INV6_N2]
  Medidor18/1(Med_n2) -> [CT_02_BT]
  HG.1-CT.2-INV.05/1(m) -> Terminator/1
  HG.1-CT.2-INV.03/1(m) -> Terminator1/1
  HG.1-CT.2-INV.04/1(m) -> Terminator2/1
  HG.1-CT.2-INV.01/1(m) -> Terminator3/1
  HG.1-CT.2-INV.02/1(m) -> Terminator4/1
  HG.1-CT.2-INV.06/1(m) -> Terminator5/1
  HG.1-CT.2-INV.07/1(m) -> Terminator6/1
  HG.1-CT.2-INV.08/1(m) -> Terminator7/1
  HG.1-CT.2-INV.09/1(m) -> Terminator8/1
  Q_ref/1 -> [Q_ref_CT2]
  [Q_ref_CT2] -> Mux1/2
  [P_ct2_inv01] -> Mux1/1
  Mux1/1 -> HG.1-CT.2-INV.03/1(PQ)
  [P_ct2_inv01] -> Mux2/1
  [Q_ref_CT2] -> Mux2/2
  Mux2/1 -> HG.1-CT.2-INV.04/1(PQ)
  Mux3/1 -> HG.1-CT.2-INV.01/1(PQ)
  [Q_ref_CT2] -> Mux3/2
  [P_ct2_inv01] -> Mux3/1
  [P_ct2_inv01] -> Mux4/1
  [Q_ref_CT2] -> Mux4/2
  Mux4/1 -> HG.1-CT.2-INV.02/1(PQ)
  Mux5/1 -> HG.1-CT.2-INV.07/1(PQ)
  [P_ct2_inv01] -> Mux5/1
  [Q_ref_CT2] -> Mux5/2
  [Q_ref_CT2] -> Mux8/2
  [P_ct2_inv01] -> Mux8/1
  Mux8/1 -> HG.1-CT.2-INV.08/1(PQ)
  Mux9/1 -> HG.1-CT.2-INV.09/1(PQ)
  [P_ct2_inv01] -> Mux9/1
  [Q_ref_CT2] -> Mux9/2
  connections:
  Medidor18/LConn1 -- A/RConn1
  Medidor18/LConn2 -- B/RConn1
  HG.1_CT.2-INV.06/RConn2 -- HG.1-CT.2-INV.06/RConn2
  HG.1_CT.2-INV.01/RConn2 -- HG.1-CT.2-INV.01/RConn2
  HG.1_CT.2-INV.06/LConn2 -- CT.02-INV.6-N2/RConn2
  HG.1_CT.2-INV.08/RConn2 -- HG.1-CT.2-INV.08/RConn2
  HG.1_CT.2-INV.07/RConn3 -- HG.1-CT.2-INV.07/RConn3
  HG.1_CT.2-INV.05/LConn2 -- CT.02-INV.5-N2/RConn2
  HG.1_CT.2-INV.01/LConn1 -- CT.02-INV.1-N2/RConn1
  HG.1_CT.2-INV.02/LConn1 -- CT.02-INV.2-N2/RConn1
  HG.1_CT.2-INV.01/RConn1 -- HG.1-CT.2-INV.01/RConn1
  HG.1_CT.2-INV.04/RConn2 -- HG.1-CT.2-INV.04/RConn2
  HG.1_CT.2-INV.05/RConn3 -- HG.1-CT.2-INV.05/RConn3
  HG.1_CT.2-INV.04/LConn2 -- CT.02-INV.4-N2/RConn2
  HG.1_CT.2-INV.09/LConn2 -- CT.02-INV.9-N2/RConn2
  HG.1_CT.2-INV.06/RConn1 -- HG.1-CT.2-INV.06/RConn1
  HG.1_CT.2-INV.03/LConn1 -- CT.02-INV.3-N2/RConn1
  HG.1_CT.2-INV.04/LConn3 -- CT.02-INV.4-N2/RConn3
  HG.1_CT.2-INV.01/LConn3 -- CT.02-INV.1-N2/RConn3
  HG.1_CT.2-INV.09/RConn1 -- HG.1-CT.2-INV.09/RConn1
  CT.02-INV.4-N2/LConn3 -- CT.02-INV.2-N2/LConn3 -- CT.02-INV.9-N2/LConn3 -- CT.02-INV.1-N2/LConn3 -- CT.02-INV.8-N2/LConn3 -- CT.02-INV.3-N2/LConn3 -- CT.02-INV.7-N2/LConn3 -- CT.02-INV.5-N2/LConn3 -- CT.02-INV.6-N2/LConn3 -- Medidor18/RConn3
  CT.02-INV.3-N2/LConn2 -- CT.02-INV.4-N2/LConn2 -- CT.02-INV.8-N2/LConn2 -- CT.02-INV.1-N2/LConn2 -- CT.02-INV.2-N2/LConn2 -- CT.02-INV.9-N2/LConn2 -- CT.02-INV.7-N2/LConn2 -- CT.02-INV.5-N2/LConn2 -- CT.02-INV.6-N2/LConn2 -- Medidor18/RConn2
  HG.1_CT.2-INV.01/RConn3 -- HG.1-CT.2-INV.01/RConn3
  HG.1_CT.2-INV.08/LConn1 -- CT.02-INV.8-N2/RConn1
  HG.1_CT.2-INV.08/LConn3 -- CT.02-INV.8-N2/RConn3
  HG.1_CT.2-INV.07/LConn2 -- CT.02-INV.7-N2/RConn2
  HG.1_CT.2-INV.05/LConn1 -- CT.02-INV.5-N2/RConn1
  Medidor18/RConn1 -- CT.02-INV.6-N2/LConn1 -- CT.02-INV.2-N2/LConn1 -- CT.02-INV.9-N2/LConn1 -- CT.02-INV.1-N2/LConn1 -- CT.02-INV.8-N2/LConn1 -- CT.02-INV.4-N2/LConn1 -- CT.02-INV.3-N2/LConn1 -- CT.02-INV.7-N2/LConn1 -- CT.02-INV.5-N2/LConn1
  HG.1_CT.2-INV.07/RConn2 -- HG.1-CT.2-INV.07/RConn2
  HG.1_CT.2-INV.07/LConn3 -- CT.02-INV.7-N2/RConn3
  HG.1_CT.2-INV.09/RConn3 -- HG.1-CT.2-INV.09/RConn3
  HG.1_CT.2-INV.01/LConn2 -- CT.02-INV.1-N2/RConn2
  HG.1_CT.2-INV.03/RConn3 -- HG.1-CT.2-INV.03/RConn3
  HG.1_CT.2-INV.09/RConn2 -- HG.1-CT.2-INV.09/RConn2
  HG.1_CT.2-INV.04/RConn3 -- HG.1-CT.2-INV.04/RConn3
  HG.1_CT.2-INV.04/RConn1 -- HG.1-CT.2-INV.04/RConn1
  HG.1_CT.2-INV.03/LConn2 -- CT.02-INV.3-N2/RConn2
  HG.1_CT.2-INV.02/LConn2 -- CT.02-INV.2-N2/RConn2
  HG.1_CT.2-INV.02/RConn3 -- HG.1-CT.2-INV.02/RConn3
  HG.1_CT.2-INV.02/RConn1 -- HG.1-CT.2-INV.02/RConn1
  HG.1_CT.2-INV.03/RConn1 -- HG.1-CT.2-INV.03/RConn1
  HG.1_CT.2-INV.05/RConn2 -- HG.1-CT.2-INV.05/RConn2
  HG.1_CT.2-INV.08/LConn2 -- CT.02-INV.8-N2/RConn2
  HG.1_CT.2-INV.09/LConn3 -- CT.02-INV.9-N2/RConn3
  Medidor18/LConn3 -- C/RConn1
  HG.1_CT.2-INV.03/LConn3 -- CT.02-INV.3-N2/RConn3
  HG.1_CT.2-INV.05/RConn1 -- HG.1-CT.2-INV.05/RConn1
  HG.1_CT.2-INV.03/RConn2 -- HG.1-CT.2-INV.03/RConn2
  HG.1_CT.2-INV.05/LConn3 -- CT.02-INV.5-N2/RConn3
  HG.1_CT.2-INV.07/LConn1 -- CT.02-INV.7-N2/RConn1
  HG.1_CT.2-INV.02/LConn3 -- CT.02-INV.2-N2/RConn3
  HG.1_CT.2-INV.08/RConn1 -- HG.1-CT.2-INV.08/RConn1
  HG.1_CT.2-INV.06/LConn1 -- CT.02-INV.6-N2/RConn1
  HG.1_CT.2-INV.06/RConn3 -- HG.1-CT.2-INV.06/RConn3
  HG.1_CT.2-INV.04/LConn1 -- CT.02-INV.4-N2/RConn1
  HG.1_CT.2-INV.02/RConn2 -- HG.1-CT.2-INV.02/RConn2
  HG.1_CT.2-INV.08/RConn3 -- HG.1-CT.2-INV.08/RConn3
  HG.1_CT.2-INV.06/LConn3 -- CT.02-INV.6-N2/RConn3
  HG.1_CT.2-INV.07/RConn1 -- HG.1-CT.2-INV.07/RConn1
  HG.1_CT.2-INV.09/LConn1 -- CT.02-INV.9-N2/RConn1

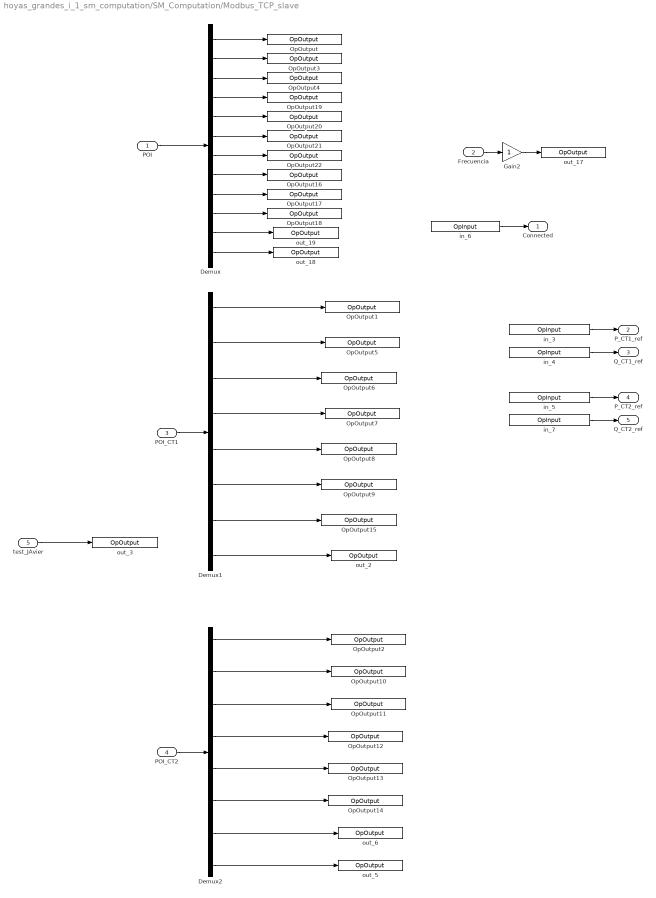
== system hoyas_grandes_i_1_sm_computation/SM_Computation/Modbus_TCP_slave ==
  POI : Inport
  Frecuencia : Inport  Port=2
  POI_CT1 : Inport  Port=3
  POI_CT2 : Inport  Port=4
  test_JAvier : Inport  Port=5
  Demux : Demux  Outputs=12
  Demux1 : Demux  Outputs=8
  Demux2 : Demux  Outputs=8
  Gain2 : Gain
  OpOutput : rtlab/OpOutput  identifier_use=POI_Vab  identifier_hide=POI_Vab  nb_parents_identifier=0
      settings: SourceProductName=RT-LAB
  OpOutput1 : rtlab/OpOutput  identifier_use=CT1_Vab  identifier_hide=CT1_Vab  nb_parents_identifier=0
      settings: SourceProductName=RT-LAB
  OpOutput10 : rtlab/OpOutput  identifier_use=CT2_Vbc  identifier_hide=CT2_Vbc  nb_parents_identifier=0
      settings: SourceProductName=RT-LAB
  OpOutput11 : rtlab/OpOutput  identifier_use=CT2_Vca  identifier_hide=CT2_Vca  nb_parents_identifier=0
      settings: SourceProductName=RT-LAB
  OpOutput12 : rtlab/OpOutput  identifier_use=CT2_Ia  identifier_hide=CT2_Ia  nb_parents_identifier=0
      settings: SourceProductName=RT-LAB
  OpOutput13 : rtlab/OpOutput  identifier_use=CT2_Ib  identifier_hide=CT2_Ib  nb_parents_identifier=0
      settings: SourceProductName=RT-LAB
  OpOutput14 : rtlab/OpOutput  identifier_use=CT2_Ic  identifier_hide=CT2_Ic  nb_parents_identifier=0
      settings: SourceProductName=RT-LAB
  OpOutput15 : rtlab/OpOutput  identifier_use=CT1_P  identifier_hide=CT1_P  nb_parents_identifier=0
      settings: SourceProductName=RT-LAB
  OpOutput16 : rtlab/OpOutput  identifier_use=POI_Va  identifier_hide=POI_Va  nb_parents_identifier=0
      settings: SourceProductName=RT-LAB
  OpOutput17 : rtlab/OpOutput  identifier_use=POI_Vb  identifier_hide=POI_Vb  nb_parents_identifier=0
      settings: SourceProductName=RT-LAB
  OpOutput18 : rtlab/OpOutput  identifier_use=POI_Vc  identifier_hide=POI_Vc  nb_parents_identifier=0
      settings: SourceProductName=RT-LAB
  OpOutput19 : rtlab/OpOutput  identifier_use=POI_Ia  identifier_hide=POI_Ia  nb_parents_identifier=0
      settings: SourceProductName=RT-LAB
  OpOutput2 : rtlab/OpOutput  identifier_use=CT2_Vab  identifier_hide=CT2_Vab  nb_parents_identifier=0
      settings: SourceProductName=RT-LAB
  OpOutput20 : rtlab/OpOutput  identifier_use=POI_Ib  identifier_hide=POI_Ib  nb_parents_identifier=0
      settings: SourceProductName=RT-LAB
  OpOutput21 : rtlab/OpOutput  identifier_use=POI_Ic  identifier_hide=POI_Ic  nb_parents_identifier=0
      settings: SourceProductName=RT-LAB
  OpOutput22 : rtlab/OpOutput  identifier_use=POI_In  identifier_hide=POI_In  nb_parents_identifier=0
      settings: SourceProductName=RT-LAB
  OpOutput3 : rtlab/OpOutput  identifier_use=POI_Vbc  identifier_hide=POI_Vbc  nb_parents_identifier=0
      settings: SourceProductName=RT-LAB
  OpOutput4 : rtlab/OpOutput  identifier_use=POI_Vca  identifier_hide=POI_Vca  nb_parents_identifier=0
      settings: SourceProductName=RT-LAB
  OpOutput5 : rtlab/OpOutput  identifier_use=CT1_Vbc  identifier_hide=CT1_Vbc  nb_parents_identifier=0
      settings: SourceProductName=RT-LAB
  OpOutput6 : rtlab/OpOutput  identifier_use=CT1_Vca  identifier_hide=CT1_Vca  nb_parents_identifier=0
      settings: SourceProductName=RT-LAB
  OpOutput7 : rtlab/OpOutput  identifier_use=CT1_Ia  identifier_hide=CT1_Ia  nb_parents_identifier=0
      settings: SourceProductName=RT-LAB
  OpOutput8 : rtlab/OpOutput  identifier_use=CT1_Ib  identifier_hide=CT1_Ib  nb_parents_identifier=0
      settings: SourceProductName=RT-LAB
  OpOutput9 : rtlab/OpOutput  identifier_use=CT1_Ic  identifier_hide=CT1_Ic  nb_parents_identifier=0
      settings: SourceProductName=RT-LAB
  in_3 : rtlab/OpInput  identifier_use=P_CT1_ref  identifier_hide=P_CT1_ref  nb_parents_identifier=0  passthrough=off  init_value=0  value_type=double  create_alias=on
      settings: SourceProductName=RT-LAB
  in_4 : rtlab/OpInput  identifier_use=Q_CT1_ref  identifier_hide=Q_CT1_ref  nb_parents_identifier=0  passthrough=off  init_value=0  value_type=double  create_alias=on
      settings: SourceProductName=RT-LAB
  in_5 : rtlab/OpInput  identifier_use=P_CT2_ref  identifier_hide=P_CT2_ref  nb_parents_identifier=0  passthrough=off  init_value=0  value_type=double  create_alias=on
      settings: SourceProductName=RT-LAB
  in_6 : rtlab/OpInput  identifier_use=Connected  identifier_hide=Connected  nb_parents_identifier=0  passthrough=off  init_value=0  value_type=double  create_alias=on
      settings: SourceProductName=RT-LAB
  in_7 : rtlab/OpInput  identifier_use=Q_CT2_ref  identifier_hide=Q_CT2_ref  nb_parents_identifier=0  passthrough=off  init_value=0  value_type=double  create_alias=on
      settings: SourceProductName=RT-LAB
  out_17 : rtlab/OpOutput  identifier_use=POI_f  identifier_hide=POI_f  nb_parents_identifier=0
      settings: SourceProductName=RT-LAB
  out_18 : rtlab/OpOutput  identifier_use=POI_Q  identifier_hide=POI_Q  nb_parents_identifier=0
      settings: SourceProductName=RT-LAB
  out_19 : rtlab/OpOutput  identifier_use=POI_P  identifier_hide=POI_P  nb_parents_identifier=0
      settings: SourceProductName=RT-LAB
  out_2 : rtlab/OpOutput  identifier_use=CT1_Q  identifier_hide=CT1_Q  nb_parents_identifier=0
      settings: SourceProductName=RT-LAB
  out_3 : rtlab/OpOutput  identifier_use=POI_CT1_P  identifier_hide=POI_CT1_P  nb_parents_identifier=0
      settings: SourceProductName=RT-LAB
  out_5 : rtlab/OpOutput  identifier_use=CT2_Q  identifier_hide=CT2_Q  nb_parents_identifier=0
      settings: SourceProductName=RT-LAB
  out_6 : rtlab/OpOutput  identifier_use=CT2_P  identifier_hide=CT2_P  nb_parents_identifier=0
      settings: SourceProductName=RT-LAB
  Connected : Outport
  P_CT1_ref : Outport  Port=2
  Q_CT1_ref : Outport  Port=3
  P_CT2_ref : Outport  Port=4
  Q_CT2_ref : Outport  Port=5
  wires:
  in_6/1 -> Connected/1
  POI/1 -> Demux/1
  POI_CT1/1 -> Demux1/1
  POI_CT2/1 -> Demux2/1
  in_3/1 -> P_CT1_ref/1
  in_4/1 -> Q_CT1_ref/1
  in_7/1 -> Q_CT2_ref/1
  in_5/1 -> P_CT2_ref/1
  Frecuencia/1 -> Gain2/1
  Gain2/1 -> out_17/1
  Demux1/1 -> OpOutput1/1
  Demux1/2 -> OpOutput5/1
  Demux1/3 -> OpOutput6/1
  Demux1/8 -> out_2/1
  Demux1/7 -> OpOutput15/1
  Demux1/4 -> OpOutput7/1
  Demux1/5 -> OpOutput8/1
  Demux1/6 -> OpOutput9/1
  Demux2/1 -> OpOutput2/1
  Demux2/8 -> out_5/1
  Demux2/7 -> out_6/1
  Demux2/2 -> OpOutput10/1
  Demux2/3 -> OpOutput11/1
  Demux2/4 -> OpOutput12/1
  Demux2/5 -> OpOutput13/1
  Demux2/6 -> OpOutput14/1
  test_JAvier/1 -> out_3/1
  Demux/1 -> OpOutput/1
  Demux/2 -> OpOutput3/1
  Demux/3 -> OpOutput4/1
  Demux/4 -> OpOutput19/1
  Demux/5 -> OpOutput20/1
  Demux/6 -> OpOutput21/1
  Demux/7 -> OpOutput22/1
  Demux/8 -> OpOutput16/1
  Demux/9 -> OpOutput17/1
  Demux/10 -> OpOutput18/1
  Demux/11 -> out_19/1
  Demux/12 -> out_18/1

== system hoyas_grandes_i_1_sm_computation/SM_Computation/OpComm1 ==
  Demux : Demux  Outputs="[1  1]"
  Receive : opal_lib/Communication/OpRecPar FromNT  Data_width=2  InitialConditions=[0;1]
  busStruct : Subsystem
  Out1 : Outport
  Out2 : Outport  Port=2
  wires:
  Demux/2 -> busStruct/2(In2)
  Demux/1 -> busStruct/1(In1)
  busStruct/2(Out2) -> Out2/1
  busStruct/1(Out1) -> Out1/1
  Receive/1 -> Demux/1

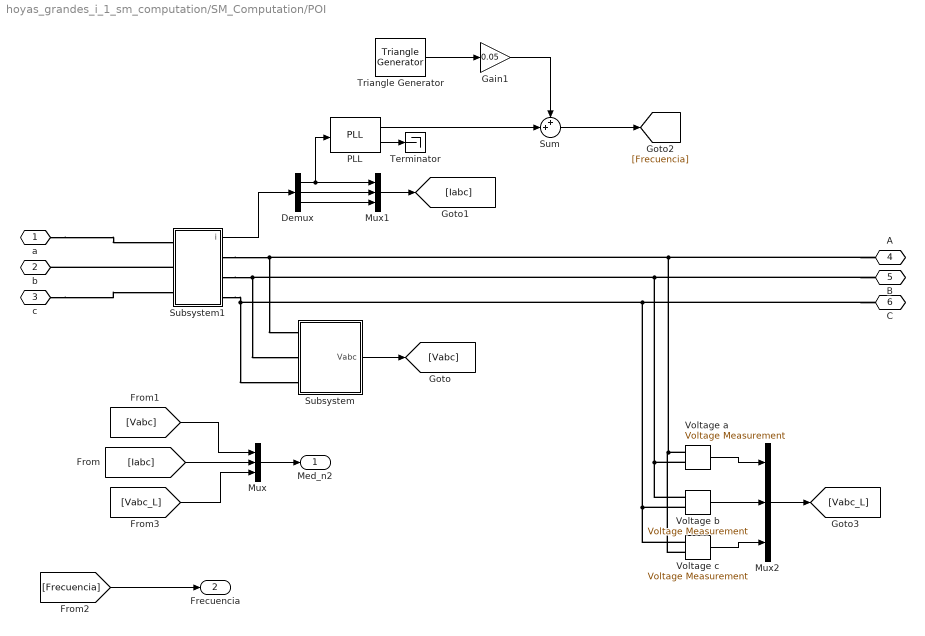
== system hoyas_grandes_i_1_sm_computation/SM_Computation/POI ==
  Demux : Demux  Outputs=3
  Gain1 : Gain  Gain=0.05
  Mux : Mux  Inputs=3
  Mux1 : Mux  Inputs=3
  Mux2 : Mux  Inputs=3
  PLL : spsPLLLib/PLL  Fmin=45  Par_Init=[0, 50]  ParK=[180, 3200, 1]  TcD=1e-4  MaxRateChangeFreq=12  FilterCutOffFreq=25  Ts=Ts_Power  AGC=on
      settings: LibrarySourceBlock=sps_lib/Control/PLL
  Subsystem : Subsystem
  Subsystem1 : Subsystem
  Sum : Sum  Inputs=++|
  Terminator : Terminator
  Triangle Generator : spsTriangleGeneratorLib/Triangle Generator  Freq=0.1  Phase=0  Ts=Ts_Power
  Voltage a : spsVoltageMeasurementLib/Voltage Measurement  PhasorSimulation=off  OutputType=Complex  PSBequivalent=0
  Voltage b : spsVoltageMeasurementLib/Voltage Measurement  PhasorSimulation=off  OutputType=Complex  PSBequivalent=0
  Voltage c : spsVoltageMeasurementLib/Voltage Measurement  PhasorSimulation=off  OutputType=Complex  PSBequivalent=0
  a : PMIOPort  Side=Right
  b : PMIOPort  Port=2  Side=Right
  c : PMIOPort  Port=3  Side=Right
  A : PMIOPort  Port=4  Side=Left
  B : PMIOPort  Port=5  Side=Left
  C : PMIOPort  Port=6  Side=Left
  Med_n2 : Outport
  Frecuencia : Outport  Port=2
  wires:
  Mux/1 -> Med_n2/1
  [Iabc] -> Mux/2
  [Vabc] -> Mux/1
  Subsystem/1(Vabc) -> [Vabc]
  Mux1/1 -> [Iabc]
  Subsystem1/1(i) -> Demux/1
  Demux/1 -> PLL/1, Mux1/1
  Demux/2 -> Mux1/2
  Demux/3 -> Mux1/3
  PLL/2 -> Terminator/1
  [Frecuencia] -> Frecuencia/1
  Sum/1 -> [Frecuencia]
  Triangle Generator/1 -> Gain1/1
  PLL/1 -> Sum/2
  Gain1/1 -> Sum/1
  Voltage a/1 -> Mux2/1
  Voltage b/1 -> Mux2/2
  Voltage c/1 -> Mux2/3
  Mux2/1 -> [Vabc_L]
  [Vabc_L] -> Mux/3
  connections:
  a/RConn1 -- Subsystem1/LConn1
  Subsystem1/LConn2 -- b/RConn1
  c/RConn1 -- Subsystem1/LConn3
  Voltage c/LConn1 -- Subsystem/LConn3 -- Subsystem1/RConn3 -- C/RConn1 -- Voltage b/LConn2
  Voltage a/LConn1 -- Subsystem/LConn1 -- Subsystem1/RConn1 -- A/RConn1 -- Voltage c/LConn2
  Voltage b/LConn1 -- Subsystem/LConn2 -- Subsystem1/RConn2 -- B/RConn1 -- Voltage a/LConn2

== system hoyas_grandes_i_1_sm_computation/SM_Computation/Subsystem1 ==
  P_profile : Inport
  P_PPC : Inport  Port=2
  PPC : Constant  Commented=on  Value=0
  Perfil : Constant  Commented=on  Value=3e3
  RTE Conversion : rteventslib/Signal Attributes/RTE Conversion  inputdatatype=RTE Boolean  outputdatatype=Double  compensation=Enabled  nbMaxEvents=10  sampleTime=Ts_Power
      settings: SourceProductName=RT-EVENTS
  RTE Relational Operator1 : rteventslib/Math Operations/RTE Relational Operator  RelationalOperator=>  NumberMaxEvents=1  SampleTime=Ts_Power
      settings: SourceProductName=RT-EVENTS
  Switch : Switch  Criteria=u2 > Threshold  SaturateOnIntegerOverflow=off  InputSameDT=off
  Out1 : Outport
  wires:
  P_profile/1 -> [Perfil]
  P_PPC/1 -> [PPC]
  RTE Relational Operator1/1 -> RTE Conversion/1
  RTE Conversion/1 -> Switch/2
  Switch/1 -> Out1/1
  [Perfil] -> Switch/3, RTE Relational Operator1/1
  [PPC] -> Switch/1, RTE Relational Operator1/2
